simulink model "SimPowerSystem_gettingstarted_07"  (Simulink 8.7)
settings: Solver=ode45  StartTime=0.0  StopTime=Inf  RelTol=1e-3
libraries: powerlib x5
settings Model: Creator=media  LastModifiedBy=media
settings DebuggingCC: UnderspecifiedInitializationDetection=Simplified  MergeDetectMultiDrivingBlocksExec=error

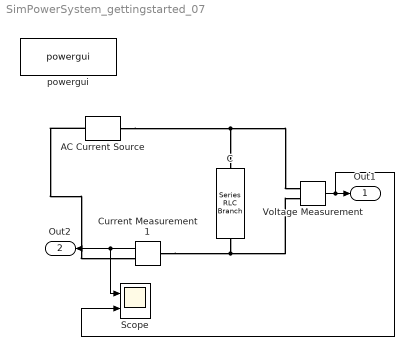
== system SimPowerSystem_gettingstarted_07 ==
  AC Current Source : powerlib/Electrical Sources/AC Current Source  Amplitude=10  Phase=0  Frequency=60  SampleTime=0  Measurements=None
  C : powerlib/Elements/Series RLC Branch  LConnTagsString=__new0  RConnTagsString=__new0  BranchType=C  Resistance=0  Inductance=0  SetiL0=off  InitialCurrent=0  Capacitance=29.5  Setx0=on  InitialVoltage=650  Measurements=None
  Current Measurement1 : powerlib/Measurements/Current Measurement  PhasorSimulation=off  OutputType=Complex  PSBequivalent=0
  Scope : Scope  NumInputPorts=2
  Voltage Measurement : powerlib/Measurements/Voltage Measurement  PhasorSimulation=off  OutputType=Complex  PSBequivalent=0
  powergui : powerlib/powergui  Priority=1  SimulationMode=Discrete  SolverType=Tustin  SampleTime=500e-9  frequency=60  SPID=off  DisableSnubberDevices=off  DisableRonSwitches=off  DisableVfSwitches=off  SwTol=0  DisplayEquations=off  Interpol=off  ExternalGateDelay=off  methode=off  Ts=100  FunctionMessages=off  echomessages=off  HookPort=off  EnableUseOfTLC=off  x0status=blocks  frequencyindice=60  Pbase=100e6  ErrMax=1e-4  Iterations=50  UnitsV=kV  UnitsW=MW  buscounter=0  RestoreLinks=warning  ResistiveCurrentMeasurement=off  Frange=[0:2:500]  Ylog=off  Xlog=on  ShowGrid=off  save=off  variable=ZData  structure=ScopeData  ZoomFFT=on  StartTime=0.0  cycles=1  DisplayStyle=2  fundamental=60  FreqAxis=off  MaxFrequency=100  frequencyindicesteady=1  RmsSteady=2  display=off
  Out1 : Outport
  Out2 : Outport  Port=2
  wires:
  Current Measurement1/1 -> Scope/1, Out2/1
  Voltage Measurement/1 -> Scope/2, Out1/1
  connections:
  Voltage Measurement/LConn1 -- AC Current Source/RConn1 -- C/LConn1
  Current Measurement1/LConn1 -- C/RConn1 -- Voltage Measurement/LConn2
  AC Current Source/LConn1 -- Current Measurement1/RConn1
